simulink model "GalvoTransferFuncFeedback"  (R2013a)
settings: Solver=ode23  StartTime=0.0  StopTime=init.StopTime  FixedStep=1e-6  MinStep=init.MinStepSize  RelTol=1e-3
undefined symbols (not defined in the file or in its folder): init, MinStepSize, TsCtrl, TsSens, TsSens2
libraries: simulink x4
settings Model: BufferReuse=off  Creator=mainster  LastModifiedBy=mainster
settings SolverCC: InitialStep=init.MinStepSize
settings DataIOCC: SignalLoggingSaveFormat=ModelDataLogs
settings OptimizationCC: OptimizeBlockIOStorage=off  BufferReuse=off  ExpressionFolding=off  ExpressionDepthLimit=2147483647  LocalBlockOutputs=off
settings DebuggingCC: FcnCallInpInsideContextMsg=UseLocalSettings
settings GRTTargetCC: CombineOutputUpdateFcns=off  GRTInterface=on

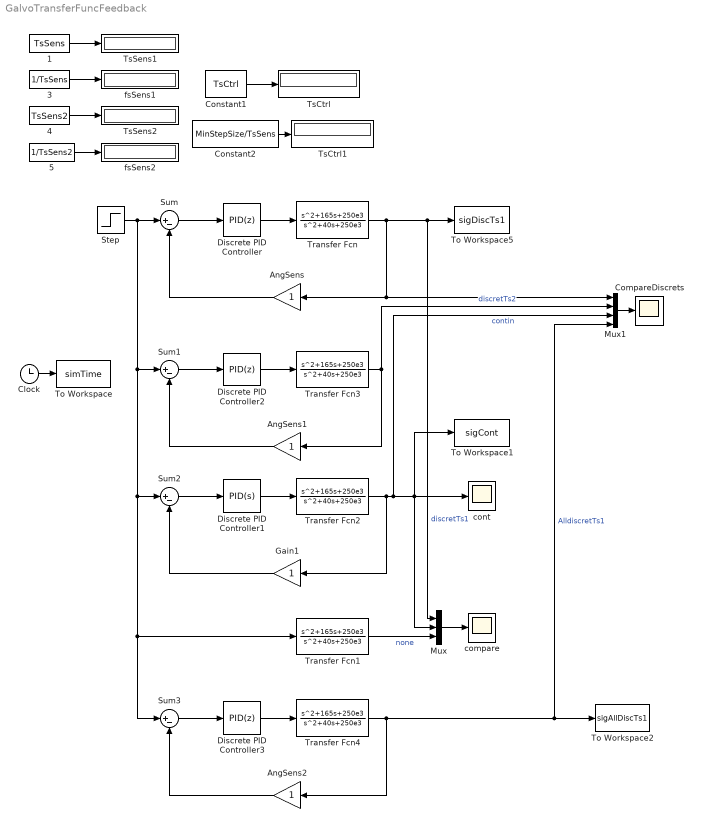
== system GalvoTransferFuncFeedback ==
  1 : Constant  Value=TsSens
  3 : Constant  Value=1/TsSens
  4 : Constant  Value=TsSens2
  5 : Constant  Value=1/TsSens2
  AngSens : Gain  SampleTime=init.TsSens
  AngSens1 : Gain  SampleTime=init.TsSens2
  AngSens2 : Gain  SampleTime=init.TsSens
  Clock : Clock
  CompareDiscrets : Scope
      settings: ShowLegends=on  TimeRange=0.05  YMin=0.9  YMax=1.1
  Constant1 : Constant  Value=TsCtrl
  Constant2 : Constant  Value=MinStepSize/TsSens
  Discrete PID Controller : simulink/Continuous/PID Controller  Controller=PID  TimeDomain=Discrete-time  SampleTime=init.TsCtrl  IntegratorMethod=Forward Euler  FilterMethod=Forward Euler  Form=Parallel  P=0.127867810268812  I=2557.35620537625  D=0  N=100  InitialConditionSource=internal  InitialConditionForIntegrator=0  InitialConditionForFilter=0  ExternalReset=none  LimitOutput=off  UpperSaturationLimit=inf  LowerSaturationLimit=-inf  LinearizeAsGain=off  AntiWindupMode=none  Kb=1  TrackingMode=off  Kt=1  PParamMin=[]  PParamMax=[]  IParamMin=[]  IParamMax=[]  DParamMin=[]  DParamMax=[]  NParamMin=[]  NParamMax=[]  KbParamMin=[]  KbParamMax=[]  KtParamMin=[]  KtParamMax=[]  POutMin=[]  POutMax=[]  IOutMin=[]  IOutMax=[]  DOutMin=[]  DOutMax=[]  NOutMin=[]  NOutMax=[]  KbOutMin=[]  KbOutMax=[]  KtOutMin=[]  KtOutMax=[]  IntegratorOutMin=[]  IntegratorOutMax=[]  FilterOutMin=[]  FilterOutMax=[]  SumOutMin=[]  SumOutMax=[]  SumI1OutMin=[]  SumI1OutMax=[]  SumI2OutMin=[]  SumI2OutMax=[]  SumI3OutMin=[]  SumI3OutMax=[]  SumDOutMin=[]  SumDOutMax=[]  SaturationOutMin=[]  SaturationOutMax=[]  IntegratorContinuousStateAttributes=''  IntegratorStateMustResolveToSignalObject=off  IntegratorRTWStateStorageClass=Auto  FilterContinuousStateAttributes=''  FilterStateMustResolveToSignalObject=off  FilterRTWStateStorageClass=Auto
  Discrete PID Controller1 : simulink/Continuous/PID Controller  Controller=PID  TimeDomain=Continuous-time  SampleTime=100e-6  IntegratorMethod=Forward Euler  FilterMethod=Forward Euler  Form=Parallel  P=0  I=3996.69881374837  D=0  N=100  InitialConditionSource=internal  InitialConditionForIntegrator=0  InitialConditionForFilter=0  ExternalReset=none  LimitOutput=off  UpperSaturationLimit=inf  LowerSaturationLimit=-inf  LinearizeAsGain=off  AntiWindupMode=none  Kb=1  TrackingMode=off  Kt=1  PParamMin=[]  PParamMax=[]  IParamMin=[]  IParamMax=[]  DParamMin=[]  DParamMax=[]  NParamMin=[]  NParamMax=[]  KbParamMin=[]  KbParamMax=[]  KtParamMin=[]  KtParamMax=[]  POutMin=[]  POutMax=[]  IOutMin=[]  IOutMax=[]  DOutMin=[]  DOutMax=[]  NOutMin=[]  NOutMax=[]  KbOutMin=[]  KbOutMax=[]  KtOutMin=[]  KtOutMax=[]  IntegratorOutMin=[]  IntegratorOutMax=[]  FilterOutMin=[]  FilterOutMax=[]  SumOutMin=[]  SumOutMax=[]  SumI1OutMin=[]  SumI1OutMax=[]  SumI2OutMin=[]  SumI2OutMax=[]  SumI3OutMin=[]  SumI3OutMax=[]  SumDOutMin=[]  SumDOutMax=[]  SaturationOutMin=[]  SaturationOutMax=[]  IntegratorContinuousStateAttributes=''  IntegratorStateMustResolveToSignalObject=off  IntegratorRTWStateStorageClass=Auto  FilterContinuousStateAttributes=''  FilterStateMustResolveToSignalObject=off  FilterRTWStateStorageClass=Auto
  Discrete PID Controller2 : simulink/Continuous/PID Controller  Controller=PID  TimeDomain=Discrete-time  SampleTime=init.TsCtrl  IntegratorMethod=Forward Euler  FilterMethod=Forward Euler  Form=Parallel  P=0.100098398930147  I=2001.96797860294  D=0  N=100  InitialConditionSource=internal  InitialConditionForIntegrator=0  InitialConditionForFilter=0  ExternalReset=none  LimitOutput=off  UpperSaturationLimit=inf  LowerSaturationLimit=-inf  LinearizeAsGain=off  AntiWindupMode=none  Kb=1  TrackingMode=off  Kt=1  PParamMin=[]  PParamMax=[]  IParamMin=[]  IParamMax=[]  DParamMin=[]  DParamMax=[]  NParamMin=[]  NParamMax=[]  KbParamMin=[]  KbParamMax=[]  KtParamMin=[]  KtParamMax=[]  POutMin=[]  POutMax=[]  IOutMin=[]  IOutMax=[]  DOutMin=[]  DOutMax=[]  NOutMin=[]  NOutMax=[]  KbOutMin=[]  KbOutMax=[]  KtOutMin=[]  KtOutMax=[]  IntegratorOutMin=[]  IntegratorOutMax=[]  FilterOutMin=[]  FilterOutMax=[]  SumOutMin=[]  SumOutMax=[]  SumI1OutMin=[]  SumI1OutMax=[]  SumI2OutMin=[]  SumI2OutMax=[]  SumI3OutMin=[]  SumI3OutMax=[]  SumDOutMin=[]  SumDOutMax=[]  SaturationOutMin=[]  SaturationOutMax=[]  IntegratorContinuousStateAttributes=''  IntegratorStateMustResolveToSignalObject=off  IntegratorRTWStateStorageClass=Auto  FilterContinuousStateAttributes=''  FilterStateMustResolveToSignalObject=off  FilterRTWStateStorageClass=Auto
  Discrete PID Controller3 : simulink/Continuous/PID Controller  Controller=PID  TimeDomain=Discrete-time  SampleTime=init.TsSens  IntegratorMethod=Forward Euler  FilterMethod=Forward Euler  Form=Parallel  P=0.127867810268812  I=2557.35620537625  D=0  N=100  InitialConditionSource=internal  InitialConditionForIntegrator=0  InitialConditionForFilter=0  ExternalReset=none  LimitOutput=off  UpperSaturationLimit=inf  LowerSaturationLimit=-inf  LinearizeAsGain=off  AntiWindupMode=none  Kb=1  TrackingMode=off  Kt=1  PParamMin=[]  PParamMax=[]  IParamMin=[]  IParamMax=[]  DParamMin=[]  DParamMax=[]  NParamMin=[]  NParamMax=[]  KbParamMin=[]  KbParamMax=[]  KtParamMin=[]  KtParamMax=[]  POutMin=[]  POutMax=[]  IOutMin=[]  IOutMax=[]  DOutMin=[]  DOutMax=[]  NOutMin=[]  NOutMax=[]  KbOutMin=[]  KbOutMax=[]  KtOutMin=[]  KtOutMax=[]  IntegratorOutMin=[]  IntegratorOutMax=[]  FilterOutMin=[]  FilterOutMax=[]  SumOutMin=[]  SumOutMax=[]  SumI1OutMin=[]  SumI1OutMax=[]  SumI2OutMin=[]  SumI2OutMax=[]  SumI3OutMin=[]  SumI3OutMax=[]  SumDOutMin=[]  SumDOutMax=[]  SaturationOutMin=[]  SaturationOutMax=[]  IntegratorContinuousStateAttributes=''  IntegratorStateMustResolveToSignalObject=off  IntegratorRTWStateStorageClass=Auto  FilterContinuousStateAttributes=''  FilterStateMustResolveToSignalObject=off  FilterRTWStateStorageClass=Auto
  Gain1 : Gain
  Mux : Mux  Inputs=3
  Mux1 : Mux
  Step : Step  Time=0.01  SampleTime=0
  Sum : Sum  Inputs=|+-  SampleTime=init.TsSens
  Sum1 : Sum  Inputs=|+-  SampleTime=init.TsSens2
  Sum2 : Sum  Inputs=|+-
  Sum3 : Sum  Inputs=|+-  SampleTime=init.TsSens
  To Workspace : ToWorkspace  VariableName=simTime  SampleTime=-1  SaveFormat=Timeseries
  To Workspace1 : ToWorkspace  VariableName=sigCont  SampleTime=-1  SaveFormat=Structure
  To Workspace2 : ToWorkspace  VariableName=sigAllDiscTs1  SampleTime=-1  SaveFormat=Structure
  To Workspace5 : ToWorkspace  VariableName=sigDiscTs1  SampleTime=-1  SaveFormat=Structure
  Transfer Fcn{,1..4} (5 alike) : TransferFcn  Numerator=[1 165 250e3]  Denominator=[1 40 250e3]
  TsCtrl : Display
      settings: Format=short_e
  TsCtrl1 : Display
      settings: Format=short_e
  TsSens1 : Display
      settings: Format=short_e
  TsSens2 : Display
      settings: Format=short_e
  compare : Scope
      settings: TickLabels=on  ShowLegends=on  TimeRange=0.05  YMin=0  YMax=1.4  SaveName=ScopeData2
  cont : Scope
  fsSens1 : Display
      settings: Format=short_e
  fsSens2 : Display
      settings: Format=short_e
  wires:
  Step/1 -> Sum/1, Sum1/1, Sum2/1, Sum3/1, Transfer Fcn1/1
  Sum/1 -> Discrete PID Controller/1
  Transfer Fcn/1 -> Mux1/1, AngSens/1, To Workspace5/1, Mux/1  "discretTs1"
  Discrete PID Controller/1 -> Transfer Fcn/1
  Sum2/1 -> Discrete PID Controller1/1
  Transfer Fcn2/1 -> Gain1/1, Mux1/3, To Workspace1/1, cont/1, Mux/2  "contin"
  Discrete PID Controller1/1 -> Transfer Fcn2/1
  Gain1/1 -> Sum2/2
  Mux/1 -> compare/1
  Transfer Fcn1/1 -> Mux/3  "none"
  AngSens/1 -> Sum/2
  Constant1/1 -> TsCtrl/1
  Sum1/1 -> Discrete PID Controller2/1
  Transfer Fcn3/1 -> Mux1/2, AngSens1/1  "discretTs2"
  Discrete PID Controller2/1 -> Transfer Fcn3/1
  AngSens1/1 -> Sum1/2
  Mux1/1 -> CompareDiscrets/1
  Constant2/1 -> TsCtrl1/1
  Clock/1 -> To Workspace/1
  1/1 -> TsSens1/1
  3/1 -> fsSens1/1
  4/1 -> TsSens2/1
  5/1 -> fsSens2/1
  Sum3/1 -> Discrete PID Controller3/1
  Transfer Fcn4/1 -> AngSens2/1, To Workspace2/1, Mux1/4  "AlldiscretTs1"
  Discrete PID Controller3/1 -> Transfer Fcn4/1
  AngSens2/1 -> Sum3/2
